simulink model "LM_TOS_0115"  (R2018b)
settings: Solver=FixedStepDiscrete  StartTime=0.0  StopTime=inf  FixedStep=0.005  RelTol=1e-3
PostLoadFcn:
  | if any(exist('dsrtsu_mdlpostloadfcn', 'file') ~= 0), dsrtsu_mdlpostloadfcn('Execute', bdroot); end
(part 2 of 4)

== system LM_TOS_0115/adapter2/HWA_TAR_OBJ_ADP/Subsystem4 ==
  <target_object_adapter> : Inport
  Bus Creator1 : BusCreator  Inputs=9  OutDataTypeStr=Bus: TARGETOBJECT  NonVirtualBus=on
  Bus Selector4 : BusSelector  OutputSignals=dis2EgoLaneCenter,TTC_f,ID_un8,Index_un8,probWithinLane_arr_f_0,probWithinLane_arr_f_1,probWithinLane_arr_f_2,probWithinLane_arr_f_3,probWithinLane_arr_f_4,probCutIn_f,probCutOut_f,overlap_f,trackingTimeWithinLane_f
  Vector Concatenate : Concatenate  NumInputs=5
  TARGRTOBJECTS_ST : Outport  OutDataTypeStr=Bus: TARGETOBJECT
  wires:
  Bus Selector4/8 -> Vector Concatenate/4  "<probWithinLane_arr_f_3>"
  Bus Selector4/11 -> Bus Creator1/7  "<probCutOut_f>"
  Bus Selector4/10 -> Bus Creator1/6  "<probCutIn_f>"
  Bus Selector4/12 -> Bus Creator1/8  "<overlap_f>"
  Bus Selector4/9 -> Vector Concatenate/5  "<probWithinLane_arr_f_4>"
  Bus Selector4/2 -> Bus Creator1/2  "<TTC_f>"
  Bus Selector4/5 -> Vector Concatenate/1  "<probWithinLane_arr_f_0>"
  <target_object_adapter>/1 -> Bus Selector4/1
  Bus Selector4/6 -> Vector Concatenate/2  "<probWithinLane_arr_f_1>"
  Bus Selector4/13 -> Bus Creator1/9  "<trackingTimeWithinLane_f>"
  Bus Selector4/1 -> Bus Creator1/1  "<dis2EgoLaneCenter>"
  Bus Selector4/7 -> Vector Concatenate/3  "<probWithinLane_arr_f_2>"
  Vector Concatenate/1 -> Bus Creator1/5
  Bus Selector4/3 -> Bus Creator1/3  "<ID_un8>"
  Bus Creator1/1 -> TARGRTOBJECTS_ST/1
  Bus Selector4/4 -> Bus Creator1/4  "<Index_un8>"

== system LM_TOS_0115/adapter2/HWA_TAR_OBJ_ADP/Subsystem5 ==
  <target_object_adapter> : Inport
  Bus Creator1 : BusCreator  Inputs=9  OutDataTypeStr=Bus: TARGETOBJECT  NonVirtualBus=on
  Bus Selector4 : BusSelector  OutputSignals=dis2EgoLaneCenter,TTC_f,ID_un8,Index_un8,probWithinLane_arr_f_0,probWithinLane_arr_f_1,probWithinLane_arr_f_2,probWithinLane_arr_f_3,probWithinLane_arr_f_4,probCutIn_f,probCutOut_f,overlap_f,trackingTimeWithinLane_f
  Vector Concatenate : Concatenate  NumInputs=5
  TARGRTOBJECTS_ST : Outport  OutDataTypeStr=Bus: TARGETOBJECT
  wires:
  Bus Selector4/4 -> Bus Creator1/4  "<Index_un8>"
  Bus Creator1/1 -> TARGRTOBJECTS_ST/1
  Bus Selector4/3 -> Bus Creator1/3  "<ID_un8>"
  Vector Concatenate/1 -> Bus Creator1/5
  Bus Selector4/7 -> Vector Concatenate/3  "<probWithinLane_arr_f_2>"
  Bus Selector4/1 -> Bus Creator1/1  "<dis2EgoLaneCenter>"
  Bus Selector4/13 -> Bus Creator1/9  "<trackingTimeWithinLane_f>"
  Bus Selector4/6 -> Vector Concatenate/2  "<probWithinLane_arr_f_1>"
  <target_object_adapter>/1 -> Bus Selector4/1
  Bus Selector4/5 -> Vector Concatenate/1  "<probWithinLane_arr_f_0>"
  Bus Selector4/2 -> Bus Creator1/2  "<TTC_f>"
  Bus Selector4/9 -> Vector Concatenate/5  "<probWithinLane_arr_f_4>"
  Bus Selector4/12 -> Bus Creator1/8  "<overlap_f>"
  Bus Selector4/10 -> Bus Creator1/6  "<probCutIn_f>"
  Bus Selector4/11 -> Bus Creator1/7  "<probCutOut_f>"
  Bus Selector4/8 -> Vector Concatenate/4  "<probWithinLane_arr_f_3>"

== system LM_TOS_0115/adapter2/HWA_TAR_OBJ_ADP/Subsystem6 ==
  <target_object_adapter> : Inport
  Bus Creator1 : BusCreator  Inputs=9  OutDataTypeStr=Bus: TARGETOBJECT  NonVirtualBus=on
  Bus Selector4 : BusSelector  OutputSignals=dis2EgoLaneCenter,TTC_f,ID_un8,Index_un8,probWithinLane_arr_f_0,probWithinLane_arr_f_1,probWithinLane_arr_f_2,probWithinLane_arr_f_3,probWithinLane_arr_f_4,probCutIn_f,probCutOut_f,overlap_f,trackingTimeWithinLane_f
  Vector Concatenate : Concatenate  NumInputs=5
  TARGRTOBJECTS_ST : Outport  OutDataTypeStr=Bus: TARGETOBJECT
  wires:
  Bus Selector4/8 -> Vector Concatenate/4  "<probWithinLane_arr_f_3>"
  Bus Selector4/11 -> Bus Creator1/7  "<probCutOut_f>"
  Bus Selector4/10 -> Bus Creator1/6  "<probCutIn_f>"
  Bus Selector4/12 -> Bus Creator1/8  "<overlap_f>"
  Bus Selector4/9 -> Vector Concatenate/5  "<probWithinLane_arr_f_4>"
  Bus Selector4/2 -> Bus Creator1/2  "<TTC_f>"
  Bus Selector4/5 -> Vector Concatenate/1  "<probWithinLane_arr_f_0>"
  <target_object_adapter>/1 -> Bus Selector4/1
  Bus Selector4/6 -> Vector Concatenate/2  "<probWithinLane_arr_f_1>"
  Bus Selector4/13 -> Bus Creator1/9  "<trackingTimeWithinLane_f>"
  Bus Selector4/1 -> Bus Creator1/1  "<dis2EgoLaneCenter>"
  Bus Selector4/7 -> Vector Concatenate/3  "<probWithinLane_arr_f_2>"
  Vector Concatenate/1 -> Bus Creator1/5
  Bus Selector4/3 -> Bus Creator1/3  "<ID_un8>"
  Bus Creator1/1 -> TARGRTOBJECTS_ST/1
  Bus Selector4/4 -> Bus Creator1/4  "<Index_un8>"

== system LM_TOS_0115/adapter2/HWA_TAR_OBJ_ADP/Subsystem7 ==
  <target_object_adapter> : Inport
  Bus Creator1 : BusCreator  Inputs=9  OutDataTypeStr=Bus: TARGETOBJECT  NonVirtualBus=on
  Bus Selector4 : BusSelector  OutputSignals=dis2EgoLaneCenter,TTC_f,ID_un8,Index_un8,probWithinLane_arr_f_0,probWithinLane_arr_f_1,probWithinLane_arr_f_2,probWithinLane_arr_f_3,probWithinLane_arr_f_4,probCutIn_f,probCutOut_f,overlap_f,trackingTimeWithinLane_f
  Vector Concatenate : Concatenate  NumInputs=5
  TARGRTOBJECTS_ST : Outport  OutDataTypeStr=Bus: TARGETOBJECT
  wires:
  Bus Selector4/4 -> Bus Creator1/4  "<Index_un8>"
  Bus Creator1/1 -> TARGRTOBJECTS_ST/1
  Bus Selector4/3 -> Bus Creator1/3  "<ID_un8>"
  Vector Concatenate/1 -> Bus Creator1/5
  Bus Selector4/7 -> Vector Concatenate/3  "<probWithinLane_arr_f_2>"
  Bus Selector4/1 -> Bus Creator1/1  "<dis2EgoLaneCenter>"
  Bus Selector4/13 -> Bus Creator1/9  "<trackingTimeWithinLane_f>"
  Bus Selector4/6 -> Vector Concatenate/2  "<probWithinLane_arr_f_1>"
  <target_object_adapter>/1 -> Bus Selector4/1
  Bus Selector4/5 -> Vector Concatenate/1  "<probWithinLane_arr_f_0>"
  Bus Selector4/2 -> Bus Creator1/2  "<TTC_f>"
  Bus Selector4/9 -> Vector Concatenate/5  "<probWithinLane_arr_f_4>"
  Bus Selector4/12 -> Bus Creator1/8  "<overlap_f>"
  Bus Selector4/10 -> Bus Creator1/6  "<probCutIn_f>"
  Bus Selector4/11 -> Bus Creator1/7  "<probCutOut_f>"
  Bus Selector4/8 -> Vector Concatenate/4  "<probWithinLane_arr_f_3>"

== system LM_TOS_0115/adapter2/HWA_TAR_OBJ_ADP/Subsystem8 ==
  <target_object_adapter> : Inport
  Bus Creator1 : BusCreator  Inputs=9  OutDataTypeStr=Bus: TARGETOBJECT  NonVirtualBus=on
  Bus Selector4 : BusSelector  OutputSignals=dis2EgoLaneCenter,TTC_f,ID_un8,Index_un8,probWithinLane_arr_f_0,probWithinLane_arr_f_1,probWithinLane_arr_f_2,probWithinLane_arr_f_3,probWithinLane_arr_f_4,probCutIn_f,probCutOut_f,overlap_f,trackingTimeWithinLane_f
  Vector Concatenate : Concatenate  NumInputs=5
  TARGRTOBJECTS_ST : Outport  OutDataTypeStr=Bus: TARGETOBJECT
  wires:
  Bus Selector4/8 -> Vector Concatenate/4  "<probWithinLane_arr_f_3>"
  Bus Selector4/11 -> Bus Creator1/7  "<probCutOut_f>"
  Bus Selector4/10 -> Bus Creator1/6  "<probCutIn_f>"
  Bus Selector4/12 -> Bus Creator1/8  "<overlap_f>"
  Bus Selector4/9 -> Vector Concatenate/5  "<probWithinLane_arr_f_4>"
  Bus Selector4/2 -> Bus Creator1/2  "<TTC_f>"
  Bus Selector4/5 -> Vector Concatenate/1  "<probWithinLane_arr_f_0>"
  <target_object_adapter>/1 -> Bus Selector4/1
  Bus Selector4/6 -> Vector Concatenate/2  "<probWithinLane_arr_f_1>"
  Bus Selector4/13 -> Bus Creator1/9  "<trackingTimeWithinLane_f>"
  Bus Selector4/1 -> Bus Creator1/1  "<dis2EgoLaneCenter>"
  Bus Selector4/7 -> Vector Concatenate/3  "<probWithinLane_arr_f_2>"
  Vector Concatenate/1 -> Bus Creator1/5
  Bus Selector4/3 -> Bus Creator1/3  "<ID_un8>"
  Bus Creator1/1 -> TARGRTOBJECTS_ST/1
  Bus Selector4/4 -> Bus Creator1/4  "<Index_un8>"

== system LM_TOS_0115/adapter2/HWA_TAR_OBJ_ADP/Subsystem9 ==
  <target_object_adapter> : Inport
  Bus Creator1 : BusCreator  Inputs=9  OutDataTypeStr=Bus: TARGETOBJECT  NonVirtualBus=on
  Bus Selector4 : BusSelector  OutputSignals=dis2EgoLaneCenter,TTC_f,ID_un8,Index_un8,probWithinLane_arr_f_0,probWithinLane_arr_f_1,probWithinLane_arr_f_2,probWithinLane_arr_f_3,probWithinLane_arr_f_4,probCutIn_f,probCutOut_f,overlap_f,trackingTimeWithinLane_f
  Vector Concatenate : Concatenate  NumInputs=5
  TARGRTOBJECTS_ST : Outport  OutDataTypeStr=Bus: TARGETOBJECT
  wires:
  Bus Selector4/4 -> Bus Creator1/4  "<Index_un8>"
  Bus Creator1/1 -> TARGRTOBJECTS_ST/1
  Bus Selector4/3 -> Bus Creator1/3  "<ID_un8>"
  Vector Concatenate/1 -> Bus Creator1/5
  Bus Selector4/7 -> Vector Concatenate/3  "<probWithinLane_arr_f_2>"
  Bus Selector4/1 -> Bus Creator1/1  "<dis2EgoLaneCenter>"
  Bus Selector4/13 -> Bus Creator1/9  "<trackingTimeWithinLane_f>"
  Bus Selector4/6 -> Vector Concatenate/2  "<probWithinLane_arr_f_1>"
  <target_object_adapter>/1 -> Bus Selector4/1
  Bus Selector4/5 -> Vector Concatenate/1  "<probWithinLane_arr_f_0>"
  Bus Selector4/2 -> Bus Creator1/2  "<TTC_f>"
  Bus Selector4/9 -> Vector Concatenate/5  "<probWithinLane_arr_f_4>"
  Bus Selector4/12 -> Bus Creator1/8  "<overlap_f>"
  Bus Selector4/10 -> Bus Creator1/6  "<probCutIn_f>"
  Bus Selector4/11 -> Bus Creator1/7  "<probCutOut_f>"
  Bus Selector4/8 -> Vector Concatenate/4  "<probWithinLane_arr_f_3>"

== system LM_TOS_0115/adapter2/Lane_0/Subsystem ==
  <LANE_0_TARGETOBJECT_0_ST> : Inport
  Bus Creator1 : BusCreator  Inputs=9  OutDataTypeStr=Bus: TARGETOBJECT  NonVirtualBus=on
  Bus Selector4 : BusSelector  OutputSignals=dis2EgoLaneCenter,TTC_f,ID_un8,Index_un8,probWithinLane_arr_f_0,probWithinLane_arr_f_1,probWithinLane_arr_f_2,probWithinLane_arr_f_3,probWithinLane_arr_f_4,probCutIn_f,probCutOut_f,overlap_f,trackingTimeWithinLane_f
  Vector Concatenate : Concatenate  NumInputs=5
  TARGRTOBJECTS_ST : Outport  OutDataTypeStr=Bus: TARGETOBJECT
  wires:
  Bus Selector4/4 -> Bus Creator1/4  "<Index_un8>"
  Bus Creator1/1 -> TARGRTOBJECTS_ST/1
  Bus Selector4/3 -> Bus Creator1/3  "<ID_un8>"
  Vector Concatenate/1 -> Bus Creator1/5
  Bus Selector4/7 -> Vector Concatenate/3  "<probWithinLane_arr_f_2>"
  Bus Selector4/1 -> Bus Creator1/1  "<dis2EgoLaneCenter>"
  Bus Selector4/13 -> Bus Creator1/9  "<trackingTimeWithinLane_f>"
  Bus Selector4/6 -> Vector Concatenate/2  "<probWithinLane_arr_f_1>"
  <LANE_0_TARGETOBJECT_0_ST>/1 -> Bus Selector4/1
  Bus Selector4/5 -> Vector Concatenate/1  "<probWithinLane_arr_f_0>"
  Bus Selector4/2 -> Bus Creator1/2  "<TTC_f>"
  Bus Selector4/9 -> Vector Concatenate/5  "<probWithinLane_arr_f_4>"
  Bus Selector4/12 -> Bus Creator1/8  "<overlap_f>"
  Bus Selector4/10 -> Bus Creator1/6  "<probCutIn_f>"
  Bus Selector4/11 -> Bus Creator1/7  "<probCutOut_f>"
  Bus Selector4/8 -> Vector Concatenate/4  "<probWithinLane_arr_f_3>"

== system LM_TOS_0115/adapter2/Lane_0/Subsystem1 ==
  <LANE_0_TARGETOBJECT_0_ST> : Inport
  Bus Creator1 : BusCreator  Inputs=9  OutDataTypeStr=Bus: TARGETOBJECT  NonVirtualBus=on
  Bus Selector4 : BusSelector  OutputSignals=dis2EgoLaneCenter,TTC_f,ID_un8,Index_un8,probWithinLane_arr_f_0,probWithinLane_arr_f_1,probWithinLane_arr_f_2,probWithinLane_arr_f_3,probWithinLane_arr_f_4,probCutIn_f,probCutOut_f,overlap_f,trackingTimeWithinLane_f
  Vector Concatenate : Concatenate  NumInputs=5
  TARGRTOBJECTS_ST : Outport  OutDataTypeStr=Bus: TARGETOBJECT
  wires:
  Bus Selector4/8 -> Vector Concatenate/4  "<probWithinLane_arr_f_3>"
  Bus Selector4/11 -> Bus Creator1/7  "<probCutOut_f>"
  Bus Selector4/10 -> Bus Creator1/6  "<probCutIn_f>"
  Bus Selector4/12 -> Bus Creator1/8  "<overlap_f>"
  Bus Selector4/9 -> Vector Concatenate/5  "<probWithinLane_arr_f_4>"
  Bus Selector4/2 -> Bus Creator1/2  "<TTC_f>"
  Bus Selector4/5 -> Vector Concatenate/1  "<probWithinLane_arr_f_0>"
  <LANE_0_TARGETOBJECT_0_ST>/1 -> Bus Selector4/1
  Bus Selector4/6 -> Vector Concatenate/2  "<probWithinLane_arr_f_1>"
  Bus Selector4/13 -> Bus Creator1/9  "<trackingTimeWithinLane_f>"
  Bus Selector4/1 -> Bus Creator1/1  "<dis2EgoLaneCenter>"
  Bus Selector4/7 -> Vector Concatenate/3  "<probWithinLane_arr_f_2>"
  Vector Concatenate/1 -> Bus Creator1/5
  Bus Selector4/3 -> Bus Creator1/3  "<ID_un8>"
  Bus Creator1/1 -> TARGRTOBJECTS_ST/1
  Bus Selector4/4 -> Bus Creator1/4  "<Index_un8>"

== system LM_TOS_0115/adapter2/Lane_0/Subsystem10 ==
  <LANE_0_TARGETOBJECT_0_ST> : Inport
  Bus Creator1 : BusCreator  Inputs=7  OutDataTypeStr=Bus: SEGMENT  NonVirtualBus=on
  Bus Selector4 : BusSelector  OutputSignals=coef_arr_f_0,coef_arr_f_1,coef_arr_f_2,coef_arr_f_3,dlowerLimit_f,dupperLimit_f,numOfSegment_un8,available_b,detectedByVideo_b,quality_f
  Vector Concatenate : Concatenate  NumInputs=4
  SEGMENT_ST : Outport  OutDataTypeStr=Bus: SEGMENT
  wires:
  Bus Creator1/1 -> SEGMENT_ST/1
  <LANE_0_TARGETOBJECT_0_ST>/1 -> Bus Selector4/1
  Bus Selector4/2 -> Vector Concatenate/2  "<coef_arr_f_1>"
  Bus Selector4/1 -> Vector Concatenate/1  "<coef_arr_f_0>"
  Bus Selector4/3 -> Vector Concatenate/3  "<coef_arr_f_2>"
  Bus Selector4/4 -> Vector Concatenate/4  "<coef_arr_f_3>"
  Vector Concatenate/1 -> Bus Creator1/1
  Bus Selector4/5 -> Bus Creator1/2  "<dlowerLimit_f>"
  Bus Selector4/10 -> Bus Creator1/7  "<quality_f>"
  Bus Selector4/9 -> Bus Creator1/6  "<detectedByVideo_b>"
  Bus Selector4/8 -> Bus Creator1/5  "<available_b>"
  Bus Selector4/7 -> Bus Creator1/4  "<numOfSegment_un8>"
  Bus Selector4/6 -> Bus Creator1/3  "<dupperLimit_f>"

== system LM_TOS_0115/adapter2/Lane_0/Subsystem11 ==
  <LANE_0_TARGETOBJECT_0_ST> : Inport
  Bus Creator1 : BusCreator  Inputs=7  OutDataTypeStr=Bus: SEGMENT  NonVirtualBus=on
  Bus Selector4 : BusSelector  OutputSignals=coef_arr_f_0,coef_arr_f_1,coef_arr_f_2,coef_arr_f_3,dlowerLimit_f,dupperLimit_f,numOfSegment_un8,available_b,detectedByVideo_b,quality_f
  Vector Concatenate : Concatenate  NumInputs=4
  SEGMENT_ST : Outport  OutDataTypeStr=Bus: SEGMENT
  wires:
  Bus Selector4/6 -> Bus Creator1/3  "<dupperLimit_f>"
  Bus Selector4/7 -> Bus Creator1/4  "<numOfSegment_un8>"
  Bus Selector4/8 -> Bus Creator1/5  "<available_b>"
  Bus Selector4/9 -> Bus Creator1/6  "<detectedByVideo_b>"
  Bus Selector4/10 -> Bus Creator1/7  "<quality_f>"
  Bus Selector4/5 -> Bus Creator1/2  "<dlowerLimit_f>"
  Vector Concatenate/1 -> Bus Creator1/1
  Bus Selector4/4 -> Vector Concatenate/4  "<coef_arr_f_3>"
  Bus Selector4/3 -> Vector Concatenate/3  "<coef_arr_f_2>"
  Bus Selector4/1 -> Vector Concatenate/1  "<coef_arr_f_0>"
  Bus Selector4/2 -> Vector Concatenate/2  "<coef_arr_f_1>"
  <LANE_0_TARGETOBJECT_0_ST>/1 -> Bus Selector4/1
  Bus Creator1/1 -> SEGMENT_ST/1

== system LM_TOS_0115/adapter2/Lane_0/Subsystem12 ==
  <LANE_0_TARGETOBJECT_0_ST> : Inport
  Bus Creator1 : BusCreator  Inputs=7  OutDataTypeStr=Bus: SEGMENT  NonVirtualBus=on
  Bus Selector4 : BusSelector  OutputSignals=coef_arr_f_0,coef_arr_f_1,coef_arr_f_2,coef_arr_f_3,dlowerLimit_f,dupperLimit_f,numOfSegment_un8,available_b,detectedByVideo_b,quality_f
  Vector Concatenate : Concatenate  NumInputs=4
  SEGMENT_ST : Outport  OutDataTypeStr=Bus: SEGMENT
  wires:
  Bus Creator1/1 -> SEGMENT_ST/1
  <LANE_0_TARGETOBJECT_0_ST>/1 -> Bus Selector4/1
  Bus Selector4/2 -> Vector Concatenate/2  "<coef_arr_f_1>"
  Bus Selector4/1 -> Vector Concatenate/1  "<coef_arr_f_0>"
  Bus Selector4/3 -> Vector Concatenate/3  "<coef_arr_f_2>"
  Bus Selector4/4 -> Vector Concatenate/4  "<coef_arr_f_3>"
  Vector Concatenate/1 -> Bus Creator1/1
  Bus Selector4/5 -> Bus Creator1/2  "<dlowerLimit_f>"
  Bus Selector4/10 -> Bus Creator1/7  "<quality_f>"
  Bus Selector4/9 -> Bus Creator1/6  "<detectedByVideo_b>"
  Bus Selector4/8 -> Bus Creator1/5  "<available_b>"
  Bus Selector4/7 -> Bus Creator1/4  "<numOfSegment_un8>"
  Bus Selector4/6 -> Bus Creator1/3  "<dupperLimit_f>"

== system LM_TOS_0115/adapter2/Lane_0/Subsystem13 ==
  <LANE_0_TARGETOBJECT_0_ST> : Inport
  Bus Creator1 : BusCreator  Inputs=7  OutDataTypeStr=Bus: SEGMENT  NonVirtualBus=on
  Bus Selector4 : BusSelector  OutputSignals=coef_arr_f_0,coef_arr_f_1,coef_arr_f_2,coef_arr_f_3,dlowerLimit_f,dupperLimit_f,numOfSegment_un8,available_b,detectedByVideo_b,quality_f
  Vector Concatenate : Concatenate  NumInputs=4
  SEGMENT_ST : Outport  OutDataTypeStr=Bus: SEGMENT
  wires:
  Bus Selector4/6 -> Bus Creator1/3  "<dupperLimit_f>"
  Bus Selector4/7 -> Bus Creator1/4  "<numOfSegment_un8>"
  Bus Selector4/8 -> Bus Creator1/5  "<available_b>"
  Bus Selector4/9 -> Bus Creator1/6  "<detectedByVideo_b>"
  Bus Selector4/10 -> Bus Creator1/7  "<quality_f>"
  Bus Selector4/5 -> Bus Creator1/2  "<dlowerLimit_f>"
  Vector Concatenate/1 -> Bus Creator1/1
  Bus Selector4/4 -> Vector Concatenate/4  "<coef_arr_f_3>"
  Bus Selector4/3 -> Vector Concatenate/3  "<coef_arr_f_2>"
  Bus Selector4/1 -> Vector Concatenate/1  "<coef_arr_f_0>"
  Bus Selector4/2 -> Vector Concatenate/2  "<coef_arr_f_1>"
  <LANE_0_TARGETOBJECT_0_ST>/1 -> Bus Selector4/1
  Bus Creator1/1 -> SEGMENT_ST/1

== system LM_TOS_0115/adapter2/Lane_0/Subsystem14 ==
  <LANE_0_TARGETOBJECT_0_ST> : Inport
  Bus Creator1 : BusCreator  Inputs=7  OutDataTypeStr=Bus: SEGMENT  NonVirtualBus=on
  Bus Selector4 : BusSelector  OutputSignals=coef_arr_f_0,coef_arr_f_1,coef_arr_f_2,coef_arr_f_3,dlowerLimit_f,dupperLimit_f,numOfSegment_un8,available_b,detectedByVideo_b,quality_f
  Vector Concatenate : Concatenate  NumInputs=4
  SEGMENT_ST : Outport  OutDataTypeStr=Bus: SEGMENT
  wires:
  Bus Creator1/1 -> SEGMENT_ST/1
  <LANE_0_TARGETOBJECT_0_ST>/1 -> Bus Selector4/1
  Bus Selector4/2 -> Vector Concatenate/2  "<coef_arr_f_1>"
  Bus Selector4/1 -> Vector Concatenate/1  "<coef_arr_f_0>"
  Bus Selector4/3 -> Vector Concatenate/3  "<coef_arr_f_2>"
  Bus Selector4/4 -> Vector Concatenate/4  "<coef_arr_f_3>"
  Vector Concatenate/1 -> Bus Creator1/1
  Bus Selector4/5 -> Bus Creator1/2  "<dlowerLimit_f>"
  Bus Selector4/10 -> Bus Creator1/7  "<quality_f>"
  Bus Selector4/9 -> Bus Creator1/6  "<detectedByVideo_b>"
  Bus Selector4/8 -> Bus Creator1/5  "<available_b>"
  Bus Selector4/7 -> Bus Creator1/4  "<numOfSegment_un8>"
  Bus Selector4/6 -> Bus Creator1/3  "<dupperLimit_f>"

== system LM_TOS_0115/adapter2/Lane_0/Subsystem15 ==
  <LANE_0_TARGETOBJECT_0_ST> : Inport
  Bus Creator1 : BusCreator  Inputs=7  OutDataTypeStr=Bus: SEGMENT  NonVirtualBus=on
  Bus Selector4 : BusSelector  OutputSignals=coef_arr_f_0,coef_arr_f_1,coef_arr_f_2,coef_arr_f_3,dlowerLimit_f,dupperLimit_f,numOfSegment_un8,available_b,detectedByVideo_b,quality_f
  Vector Concatenate : Concatenate  NumInputs=4
  SEGMENT_ST : Outport  OutDataTypeStr=Bus: SEGMENT
  wires:
  Bus Selector4/6 -> Bus Creator1/3  "<dupperLimit_f>"
  Bus Selector4/7 -> Bus Creator1/4  "<numOfSegment_un8>"
  Bus Selector4/8 -> Bus Creator1/5  "<available_b>"
  Bus Selector4/9 -> Bus Creator1/6  "<detectedByVideo_b>"
  Bus Selector4/10 -> Bus Creator1/7  "<quality_f>"
  Bus Selector4/5 -> Bus Creator1/2  "<dlowerLimit_f>"
  Vector Concatenate/1 -> Bus Creator1/1
  Bus Selector4/4 -> Vector Concatenate/4  "<coef_arr_f_3>"
  Bus Selector4/3 -> Vector Concatenate/3  "<coef_arr_f_2>"
  Bus Selector4/1 -> Vector Concatenate/1  "<coef_arr_f_0>"
  Bus Selector4/2 -> Vector Concatenate/2  "<coef_arr_f_1>"
  <LANE_0_TARGETOBJECT_0_ST>/1 -> Bus Selector4/1
  Bus Creator1/1 -> SEGMENT_ST/1

== system LM_TOS_0115/adapter2/Lane_0/Subsystem2 ==
  <LANE_0_TARGETOBJECT_0_ST> : Inport
  Bus Creator1 : BusCreator  Inputs=9  OutDataTypeStr=Bus: TARGETOBJECT  NonVirtualBus=on
  Bus Selector4 : BusSelector  OutputSignals=dis2EgoLaneCenter,TTC_f,ID_un8,Index_un8,probWithinLane_arr_f_0,probWithinLane_arr_f_1,probWithinLane_arr_f_2,probWithinLane_arr_f_3,probWithinLane_arr_f_4,probCutIn_f,probCutOut_f,overlap_f,trackingTimeWithinLane_f
  Vector Concatenate : Concatenate  NumInputs=5
  TARGRTOBJECTS_ST : Outport  OutDataTypeStr=Bus: TARGETOBJECT
  wires:
  Bus Selector4/4 -> Bus Creator1/4  "<Index_un8>"
  Bus Creator1/1 -> TARGRTOBJECTS_ST/1
  Bus Selector4/3 -> Bus Creator1/3  "<ID_un8>"
  Vector Concatenate/1 -> Bus Creator1/5
  Bus Selector4/7 -> Vector Concatenate/3  "<probWithinLane_arr_f_2>"
  Bus Selector4/1 -> Bus Creator1/1  "<dis2EgoLaneCenter>"
  Bus Selector4/13 -> Bus Creator1/9  "<trackingTimeWithinLane_f>"
  Bus Selector4/6 -> Vector Concatenate/2  "<probWithinLane_arr_f_1>"
  <LANE_0_TARGETOBJECT_0_ST>/1 -> Bus Selector4/1
  Bus Selector4/5 -> Vector Concatenate/1  "<probWithinLane_arr_f_0>"
  Bus Selector4/2 -> Bus Creator1/2  "<TTC_f>"
  Bus Selector4/9 -> Vector Concatenate/5  "<probWithinLane_arr_f_4>"
  Bus Selector4/12 -> Bus Creator1/8  "<overlap_f>"
  Bus Selector4/10 -> Bus Creator1/6  "<probCutIn_f>"
  Bus Selector4/11 -> Bus Creator1/7  "<probCutOut_f>"
  Bus Selector4/8 -> Vector Concatenate/4  "<probWithinLane_arr_f_3>"

== system LM_TOS_0115/adapter2/Lane_0/Subsystem3 ==
  <LANE_0_TARGETOBJECT_0_ST> : Inport
  Bus Creator1 : BusCreator  Inputs=9  OutDataTypeStr=Bus: TARGETOBJECT  NonVirtualBus=on
  Bus Selector4 : BusSelector  OutputSignals=dis2EgoLaneCenter,TTC_f,ID_un8,Index_un8,probWithinLane_arr_f_0,probWithinLane_arr_f_1,probWithinLane_arr_f_2,probWithinLane_arr_f_3,probWithinLane_arr_f_4,probCutIn_f,probCutOut_f,overlap_f,trackingTimeWithinLane_f
  Vector Concatenate : Concatenate  NumInputs=5
  TARGRTOBJECTS_ST : Outport  OutDataTypeStr=Bus: TARGETOBJECT
  wires:
  Bus Selector4/8 -> Vector Concatenate/4  "<probWithinLane_arr_f_3>"
  Bus Selector4/11 -> Bus Creator1/7  "<probCutOut_f>"
  Bus Selector4/10 -> Bus Creator1/6  "<probCutIn_f>"
  Bus Selector4/12 -> Bus Creator1/8  "<overlap_f>"
  Bus Selector4/9 -> Vector Concatenate/5  "<probWithinLane_arr_f_4>"
  Bus Selector4/2 -> Bus Creator1/2  "<TTC_f>"
  Bus Selector4/5 -> Vector Concatenate/1  "<probWithinLane_arr_f_0>"
  <LANE_0_TARGETOBJECT_0_ST>/1 -> Bus Selector4/1
  Bus Selector4/6 -> Vector Concatenate/2  "<probWithinLane_arr_f_1>"
  Bus Selector4/13 -> Bus Creator1/9  "<trackingTimeWithinLane_f>"
  Bus Selector4/1 -> Bus Creator1/1  "<dis2EgoLaneCenter>"
  Bus Selector4/7 -> Vector Concatenate/3  "<probWithinLane_arr_f_2>"
  Vector Concatenate/1 -> Bus Creator1/5
  Bus Selector4/3 -> Bus Creator1/3  "<ID_un8>"
  Bus Creator1/1 -> TARGRTOBJECTS_ST/1
  Bus Selector4/4 -> Bus Creator1/4  "<Index_un8>"

== system LM_TOS_0115/adapter2/Lane_0/Subsystem4 ==
  <LANE_0_TARGETOBJECT_0_ST> : Inport
  Bus Creator1 : BusCreator  Inputs=9  OutDataTypeStr=Bus: TARGETOBJECT  NonVirtualBus=on
  Bus Selector4 : BusSelector  OutputSignals=dis2EgoLaneCenter,TTC_f,ID_un8,Index_un8,probWithinLane_arr_f_0,probWithinLane_arr_f_1,probWithinLane_arr_f_2,probWithinLane_arr_f_3,probWithinLane_arr_f_4,probCutIn_f,probCutOut_f,overlap_f,trackingTimeWithinLane_f
  Vector Concatenate : Concatenate  NumInputs=5
  TARGRTOBJECTS_ST : Outport  OutDataTypeStr=Bus: TARGETOBJECT
  wires:
  Bus Selector4/4 -> Bus Creator1/4  "<Index_un8>"
  Bus Creator1/1 -> TARGRTOBJECTS_ST/1
  Bus Selector4/3 -> Bus Creator1/3  "<ID_un8>"
  Vector Concatenate/1 -> Bus Creator1/5
  Bus Selector4/7 -> Vector Concatenate/3  "<probWithinLane_arr_f_2>"
  Bus Selector4/1 -> Bus Creator1/1  "<dis2EgoLaneCenter>"
  Bus Selector4/13 -> Bus Creator1/9  "<trackingTimeWithinLane_f>"
  Bus Selector4/6 -> Vector Concatenate/2  "<probWithinLane_arr_f_1>"
  <LANE_0_TARGETOBJECT_0_ST>/1 -> Bus Selector4/1
  Bus Selector4/5 -> Vector Concatenate/1  "<probWithinLane_arr_f_0>"
  Bus Selector4/2 -> Bus Creator1/2  "<TTC_f>"
  Bus Selector4/9 -> Vector Concatenate/5  "<probWithinLane_arr_f_4>"
  Bus Selector4/12 -> Bus Creator1/8  "<overlap_f>"
  Bus Selector4/10 -> Bus Creator1/6  "<probCutIn_f>"
  Bus Selector4/11 -> Bus Creator1/7  "<probCutOut_f>"
  Bus Selector4/8 -> Vector Concatenate/4  "<probWithinLane_arr_f_3>"

== system LM_TOS_0115/adapter2/Lane_0/Subsystem5 ==
  <LANE_0_TARGETOBJECT_0_ST> : Inport
  Bus Creator1 : BusCreator  Inputs=9  OutDataTypeStr=Bus: TARGETOBJECT  NonVirtualBus=on
  Bus Selector4 : BusSelector  OutputSignals=dis2EgoLaneCenter,TTC_f,ID_un8,Index_un8,probWithinLane_arr_f_0,probWithinLane_arr_f_1,probWithinLane_arr_f_2,probWithinLane_arr_f_3,probWithinLane_arr_f_4,probCutIn_f,probCutOut_f,overlap_f,trackingTimeWithinLane_f
  Vector Concatenate : Concatenate  NumInputs=5
  TARGRTOBJECTS_ST : Outport  OutDataTypeStr=Bus: TARGETOBJECT
  wires:
  Bus Selector4/8 -> Vector Concatenate/4  "<probWithinLane_arr_f_3>"
  Bus Selector4/11 -> Bus Creator1/7  "<probCutOut_f>"
  Bus Selector4/10 -> Bus Creator1/6  "<probCutIn_f>"
  Bus Selector4/12 -> Bus Creator1/8  "<overlap_f>"
  Bus Selector4/9 -> Vector Concatenate/5  "<probWithinLane_arr_f_4>"
  Bus Selector4/2 -> Bus Creator1/2  "<TTC_f>"
  Bus Selector4/5 -> Vector Concatenate/1  "<probWithinLane_arr_f_0>"
  <LANE_0_TARGETOBJECT_0_ST>/1 -> Bus Selector4/1
  Bus Selector4/6 -> Vector Concatenate/2  "<probWithinLane_arr_f_1>"
  Bus Selector4/13 -> Bus Creator1/9  "<trackingTimeWithinLane_f>"
  Bus Selector4/1 -> Bus Creator1/1  "<dis2EgoLaneCenter>"
  Bus Selector4/7 -> Vector Concatenate/3  "<probWithinLane_arr_f_2>"
  Vector Concatenate/1 -> Bus Creator1/5
  Bus Selector4/3 -> Bus Creator1/3  "<ID_un8>"
  Bus Creator1/1 -> TARGRTOBJECTS_ST/1
  Bus Selector4/4 -> Bus Creator1/4  "<Index_un8>"

== system LM_TOS_0115/adapter2/Lane_0/Subsystem6 ==
  <LANE_0_TARGETOBJECT_0_ST> : Inport
  Bus Creator1 : BusCreator  Inputs=9  OutDataTypeStr=Bus: TARGETOBJECT  NonVirtualBus=on
  Bus Selector4 : BusSelector  OutputSignals=dis2EgoLaneCenter,TTC_f,ID_un8,Index_un8,probWithinLane_arr_f_0,probWithinLane_arr_f_1,probWithinLane_arr_f_2,probWithinLane_arr_f_3,probWithinLane_arr_f_4,probCutIn_f,probCutOut_f,overlap_f,trackingTimeWithinLane_f
  Vector Concatenate : Concatenate  NumInputs=5
  TARGRTOBJECTS_ST : Outport  OutDataTypeStr=Bus: TARGETOBJECT
  wires:
  Bus Selector4/4 -> Bus Creator1/4  "<Index_un8>"
  Bus Creator1/1 -> TARGRTOBJECTS_ST/1
  Bus Selector4/3 -> Bus Creator1/3  "<ID_un8>"
  Vector Concatenate/1 -> Bus Creator1/5
  Bus Selector4/7 -> Vector Concatenate/3  "<probWithinLane_arr_f_2>"
  Bus Selector4/1 -> Bus Creator1/1  "<dis2EgoLaneCenter>"
  Bus Selector4/13 -> Bus Creator1/9  "<trackingTimeWithinLane_f>"
  Bus Selector4/6 -> Vector Concatenate/2  "<probWithinLane_arr_f_1>"
  <LANE_0_TARGETOBJECT_0_ST>/1 -> Bus Selector4/1
  Bus Selector4/5 -> Vector Concatenate/1  "<probWithinLane_arr_f_0>"
  Bus Selector4/2 -> Bus Creator1/2  "<TTC_f>"
  Bus Selector4/9 -> Vector Concatenate/5  "<probWithinLane_arr_f_4>"
  Bus Selector4/12 -> Bus Creator1/8  "<overlap_f>"
  Bus Selector4/10 -> Bus Creator1/6  "<probCutIn_f>"
  Bus Selector4/11 -> Bus Creator1/7  "<probCutOut_f>"
  Bus Selector4/8 -> Vector Concatenate/4  "<probWithinLane_arr_f_3>"

== system LM_TOS_0115/adapter2/Lane_0/Subsystem7 ==
  <LANE_0_TARGETOBJECT_0_ST> : Inport
  Bus Creator1 : BusCreator  Inputs=9  OutDataTypeStr=Bus: TARGETOBJECT  NonVirtualBus=on
  Bus Selector4 : BusSelector  OutputSignals=dis2EgoLaneCenter,TTC_f,ID_un8,Index_un8,probWithinLane_arr_f_0,probWithinLane_arr_f_1,probWithinLane_arr_f_2,probWithinLane_arr_f_3,probWithinLane_arr_f_4,probCutIn_f,probCutOut_f,overlap_f,trackingTimeWithinLane_f
  Vector Concatenate : Concatenate  NumInputs=5
  TARGRTOBJECTS_ST : Outport  OutDataTypeStr=Bus: TARGETOBJECT
  wires:
  Bus Selector4/8 -> Vector Concatenate/4  "<probWithinLane_arr_f_3>"
  Bus Selector4/11 -> Bus Creator1/7  "<probCutOut_f>"
  Bus Selector4/10 -> Bus Creator1/6  "<probCutIn_f>"
  Bus Selector4/12 -> Bus Creator1/8  "<overlap_f>"
  Bus Selector4/9 -> Vector Concatenate/5  "<probWithinLane_arr_f_4>"
  Bus Selector4/2 -> Bus Creator1/2  "<TTC_f>"
  Bus Selector4/5 -> Vector Concatenate/1  "<probWithinLane_arr_f_0>"
  <LANE_0_TARGETOBJECT_0_ST>/1 -> Bus Selector4/1
  Bus Selector4/6 -> Vector Concatenate/2  "<probWithinLane_arr_f_1>"
  Bus Selector4/13 -> Bus Creator1/9  "<trackingTimeWithinLane_f>"
  Bus Selector4/1 -> Bus Creator1/1  "<dis2EgoLaneCenter>"
  Bus Selector4/7 -> Vector Concatenate/3  "<probWithinLane_arr_f_2>"
  Vector Concatenate/1 -> Bus Creator1/5
  Bus Selector4/3 -> Bus Creator1/3  "<ID_un8>"
  Bus Creator1/1 -> TARGRTOBJECTS_ST/1
  Bus Selector4/4 -> Bus Creator1/4  "<Index_un8>"

== system LM_TOS_0115/adapter2/Lane_0/Subsystem8 ==
  <LANE_0_TARGETOBJECT_0_ST> : Inport
  Bus Creator1 : BusCreator  Inputs=9  OutDataTypeStr=Bus: TARGETOBJECT  NonVirtualBus=on
  Bus Selector4 : BusSelector  OutputSignals=dis2EgoLaneCenter,TTC_f,ID_un8,Index_un8,probWithinLane_arr_f_0,probWithinLane_arr_f_1,probWithinLane_arr_f_2,probWithinLane_arr_f_3,probWithinLane_arr_f_4,probCutIn_f,probCutOut_f,overlap_f,trackingTimeWithinLane_f
  Vector Concatenate : Concatenate  NumInputs=5
  TARGRTOBJECTS_ST : Outport  OutDataTypeStr=Bus: TARGETOBJECT
  wires:
  Bus Selector4/4 -> Bus Creator1/4  "<Index_un8>"
  Bus Creator1/1 -> TARGRTOBJECTS_ST/1
  Bus Selector4/3 -> Bus Creator1/3  "<ID_un8>"
  Vector Concatenate/1 -> Bus Creator1/5
  Bus Selector4/7 -> Vector Concatenate/3  "<probWithinLane_arr_f_2>"
  Bus Selector4/1 -> Bus Creator1/1  "<dis2EgoLaneCenter>"
  Bus Selector4/13 -> Bus Creator1/9  "<trackingTimeWithinLane_f>"
  Bus Selector4/6 -> Vector Concatenate/2  "<probWithinLane_arr_f_1>"
  <LANE_0_TARGETOBJECT_0_ST>/1 -> Bus Selector4/1
  Bus Selector4/5 -> Vector Concatenate/1  "<probWithinLane_arr_f_0>"
  Bus Selector4/2 -> Bus Creator1/2  "<TTC_f>"
  Bus Selector4/9 -> Vector Concatenate/5  "<probWithinLane_arr_f_4>"
  Bus Selector4/12 -> Bus Creator1/8  "<overlap_f>"
  Bus Selector4/10 -> Bus Creator1/6  "<probCutIn_f>"
  Bus Selector4/11 -> Bus Creator1/7  "<probCutOut_f>"
  Bus Selector4/8 -> Vector Concatenate/4  "<probWithinLane_arr_f_3>"

== system LM_TOS_0115/adapter2/Lane_0/Subsystem9 ==
  <LANE_0_TARGETOBJECT_0_ST> : Inport
  Bus Creator1 : BusCreator  Inputs=9  OutDataTypeStr=Bus: TARGETOBJECT  NonVirtualBus=on
  Bus Selector4 : BusSelector  OutputSignals=dis2EgoLaneCenter,TTC_f,ID_un8,Index_un8,probWithinLane_arr_f_0,probWithinLane_arr_f_1,probWithinLane_arr_f_2,probWithinLane_arr_f_3,probWithinLane_arr_f_4,probCutIn_f,probCutOut_f,overlap_f,trackingTimeWithinLane_f
  Vector Concatenate : Concatenate  NumInputs=5
  TARGRTOBJECTS_ST : Outport  OutDataTypeStr=Bus: TARGETOBJECT
  wires:
  Bus Selector4/8 -> Vector Concatenate/4  "<probWithinLane_arr_f_3>"
  Bus Selector4/11 -> Bus Creator1/7  "<probCutOut_f>"
  Bus Selector4/10 -> Bus Creator1/6  "<probCutIn_f>"
  Bus Selector4/12 -> Bus Creator1/8  "<overlap_f>"
  Bus Selector4/9 -> Vector Concatenate/5  "<probWithinLane_arr_f_4>"
  Bus Selector4/2 -> Bus Creator1/2  "<TTC_f>"
  Bus Selector4/5 -> Vector Concatenate/1  "<probWithinLane_arr_f_0>"
  <LANE_0_TARGETOBJECT_0_ST>/1 -> Bus Selector4/1
  Bus Selector4/6 -> Vector Concatenate/2  "<probWithinLane_arr_f_1>"
  Bus Selector4/13 -> Bus Creator1/9  "<trackingTimeWithinLane_f>"
  Bus Selector4/1 -> Bus Creator1/1  "<dis2EgoLaneCenter>"
  Bus Selector4/7 -> Vector Concatenate/3  "<probWithinLane_arr_f_2>"
  Vector Concatenate/1 -> Bus Creator1/5
  Bus Selector4/3 -> Bus Creator1/3  "<ID_un8>"
  Bus Creator1/1 -> TARGRTOBJECTS_ST/1
  Bus Selector4/4 -> Bus Creator1/4  "<Index_un8>"

== system LM_TOS_0115/adapter2/Lane_1/Subsystem ==
  <LANE_1_TARGETOBJECT_0_ST> : Inport
  Bus Creator1 : BusCreator  Inputs=9  OutDataTypeStr=Bus: TARGETOBJECT  NonVirtualBus=on
  Bus Selector4 : BusSelector  OutputSignals=dis2EgoLaneCenter,TTC_f,ID_un8,Index_un8,probWithinLane_arr_f_0,probWithinLane_arr_f_1,probWithinLane_arr_f_2,probWithinLane_arr_f_3,probWithinLane_arr_f_4,probCutIn_f,probCutOut_f,overlap_f,trackingTimeWithinLane_f
  Vector Concatenate : Concatenate  NumInputs=5
  TARGRTOBJECTS_ST : Outport  OutDataTypeStr=Bus: TARGETOBJECT
  wires:
  Bus Selector4/8 -> Vector Concatenate/4  "<probWithinLane_arr_f_3>"
  Bus Selector4/11 -> Bus Creator1/7  "<probCutOut_f>"
  Bus Selector4/10 -> Bus Creator1/6  "<probCutIn_f>"
  Bus Selector4/12 -> Bus Creator1/8  "<overlap_f>"
  Bus Selector4/9 -> Vector Concatenate/5  "<probWithinLane_arr_f_4>"
  Bus Selector4/2 -> Bus Creator1/2  "<TTC_f>"
  Bus Selector4/5 -> Vector Concatenate/1  "<probWithinLane_arr_f_0>"
  <LANE_1_TARGETOBJECT_0_ST>/1 -> Bus Selector4/1
  Bus Selector4/6 -> Vector Concatenate/2  "<probWithinLane_arr_f_1>"
  Bus Selector4/13 -> Bus Creator1/9  "<trackingTimeWithinLane_f>"
  Bus Selector4/1 -> Bus Creator1/1  "<dis2EgoLaneCenter>"
  Bus Selector4/7 -> Vector Concatenate/3  "<probWithinLane_arr_f_2>"
  Vector Concatenate/1 -> Bus Creator1/5
  Bus Selector4/3 -> Bus Creator1/3  "<ID_un8>"
  Bus Creator1/1 -> TARGRTOBJECTS_ST/1
  Bus Selector4/4 -> Bus Creator1/4  "<Index_un8>"

== system LM_TOS_0115/adapter2/Lane_1/Subsystem1 ==
  <LANE_1_TARGETOBJECT_0_ST> : Inport
  Bus Creator1 : BusCreator  Inputs=9  OutDataTypeStr=Bus: TARGETOBJECT  NonVirtualBus=on
  Bus Selector4 : BusSelector  OutputSignals=dis2EgoLaneCenter,TTC_f,ID_un8,Index_un8,probWithinLane_arr_f_0,probWithinLane_arr_f_1,probWithinLane_arr_f_2,probWithinLane_arr_f_3,probWithinLane_arr_f_4,probCutIn_f,probCutOut_f,overlap_f,trackingTimeWithinLane_f
  Vector Concatenate : Concatenate  NumInputs=5
  TARGRTOBJECTS_ST : Outport  OutDataTypeStr=Bus: TARGETOBJECT
  wires:
  Bus Selector4/4 -> Bus Creator1/4  "<Index_un8>"
  Bus Creator1/1 -> TARGRTOBJECTS_ST/1
  Bus Selector4/3 -> Bus Creator1/3  "<ID_un8>"
  Vector Concatenate/1 -> Bus Creator1/5
  Bus Selector4/7 -> Vector Concatenate/3  "<probWithinLane_arr_f_2>"
  Bus Selector4/1 -> Bus Creator1/1  "<dis2EgoLaneCenter>"
  Bus Selector4/13 -> Bus Creator1/9  "<trackingTimeWithinLane_f>"
  Bus Selector4/6 -> Vector Concatenate/2  "<probWithinLane_arr_f_1>"
  <LANE_1_TARGETOBJECT_0_ST>/1 -> Bus Selector4/1
  Bus Selector4/5 -> Vector Concatenate/1  "<probWithinLane_arr_f_0>"
  Bus Selector4/2 -> Bus Creator1/2  "<TTC_f>"
  Bus Selector4/9 -> Vector Concatenate/5  "<probWithinLane_arr_f_4>"
  Bus Selector4/12 -> Bus Creator1/8  "<overlap_f>"
  Bus Selector4/10 -> Bus Creator1/6  "<probCutIn_f>"
  Bus Selector4/11 -> Bus Creator1/7  "<probCutOut_f>"
  Bus Selector4/8 -> Vector Concatenate/4  "<probWithinLane_arr_f_3>"

== system LM_TOS_0115/adapter2/Lane_1/Subsystem10 ==
  <LANE_1_TARGETOBJECT_0_ST> : Inport
  Bus Creator1 : BusCreator  Inputs=7  OutDataTypeStr=Bus: SEGMENT  NonVirtualBus=on
  Bus Selector4 : BusSelector  OutputSignals=coef_arr_f_0,coef_arr_f_1,coef_arr_f_2,coef_arr_f_3,dlowerLimit_f,dupperLimit_f,numOfSegment_un8,available_b,detectedByVideo_b,quality_f
  Vector Concatenate : Concatenate  NumInputs=4
  SEGMENT_ST : Outport  OutDataTypeStr=Bus: SEGMENT
  wires:
  Bus Selector4/6 -> Bus Creator1/3  "<dupperLimit_f>"
  Bus Selector4/7 -> Bus Creator1/4  "<numOfSegment_un8>"
  Bus Selector4/8 -> Bus Creator1/5  "<available_b>"
  Bus Selector4/9 -> Bus Creator1/6  "<detectedByVideo_b>"
  Bus Selector4/10 -> Bus Creator1/7  "<quality_f>"
  Bus Selector4/5 -> Bus Creator1/2  "<dlowerLimit_f>"
  Vector Concatenate/1 -> Bus Creator1/1
  Bus Selector4/4 -> Vector Concatenate/4  "<coef_arr_f_3>"
  Bus Selector4/3 -> Vector Concatenate/3  "<coef_arr_f_2>"
  Bus Selector4/1 -> Vector Concatenate/1  "<coef_arr_f_0>"
  Bus Selector4/2 -> Vector Concatenate/2  "<coef_arr_f_1>"
  <LANE_1_TARGETOBJECT_0_ST>/1 -> Bus Selector4/1
  Bus Creator1/1 -> SEGMENT_ST/1

== system LM_TOS_0115/adapter2/Lane_1/Subsystem11 ==
  <LANE_1_TARGETOBJECT_0_ST> : Inport
  Bus Creator1 : BusCreator  Inputs=7  OutDataTypeStr=Bus: SEGMENT  NonVirtualBus=on
  Bus Selector4 : BusSelector  OutputSignals=coef_arr_f_0,coef_arr_f_1,coef_arr_f_2,coef_arr_f_3,dlowerLimit_f,dupperLimit_f,numOfSegment_un8,available_b,detectedByVideo_b,quality_f
  Vector Concatenate : Concatenate  NumInputs=4
  SEGMENT_ST : Outport  OutDataTypeStr=Bus: SEGMENT
  wires:
  Bus Creator1/1 -> SEGMENT_ST/1
  <LANE_1_TARGETOBJECT_0_ST>/1 -> Bus Selector4/1
  Bus Selector4/2 -> Vector Concatenate/2  "<coef_arr_f_1>"
  Bus Selector4/1 -> Vector Concatenate/1  "<coef_arr_f_0>"
  Bus Selector4/3 -> Vector Concatenate/3  "<coef_arr_f_2>"
  Bus Selector4/4 -> Vector Concatenate/4  "<coef_arr_f_3>"
  Vector Concatenate/1 -> Bus Creator1/1
  Bus Selector4/5 -> Bus Creator1/2  "<dlowerLimit_f>"
  Bus Selector4/10 -> Bus Creator1/7  "<quality_f>"
  Bus Selector4/9 -> Bus Creator1/6  "<detectedByVideo_b>"
  Bus Selector4/8 -> Bus Creator1/5  "<available_b>"
  Bus Selector4/7 -> Bus Creator1/4  "<numOfSegment_un8>"
  Bus Selector4/6 -> Bus Creator1/3  "<dupperLimit_f>"

== system LM_TOS_0115/adapter2/Lane_1/Subsystem12 ==
  <LANE_1_TARGETOBJECT_0_ST> : Inport
  Bus Creator1 : BusCreator  Inputs=7  OutDataTypeStr=Bus: SEGMENT  NonVirtualBus=on
  Bus Selector4 : BusSelector  OutputSignals=coef_arr_f_0,coef_arr_f_1,coef_arr_f_2,coef_arr_f_3,dlowerLimit_f,dupperLimit_f,numOfSegment_un8,available_b,detectedByVideo_b,quality_f
  Vector Concatenate : Concatenate  NumInputs=4
  SEGMENT_ST : Outport  OutDataTypeStr=Bus: SEGMENT
  wires:
  Bus Selector4/6 -> Bus Creator1/3  "<dupperLimit_f>"
  Bus Selector4/7 -> Bus Creator1/4  "<numOfSegment_un8>"
  Bus Selector4/8 -> Bus Creator1/5  "<available_b>"
  Bus Selector4/9 -> Bus Creator1/6  "<detectedByVideo_b>"
  Bus Selector4/10 -> Bus Creator1/7  "<quality_f>"
  Bus Selector4/5 -> Bus Creator1/2  "<dlowerLimit_f>"
  Vector Concatenate/1 -> Bus Creator1/1
  Bus Selector4/4 -> Vector Concatenate/4  "<coef_arr_f_3>"
  Bus Selector4/3 -> Vector Concatenate/3  "<coef_arr_f_2>"
  Bus Selector4/1 -> Vector Concatenate/1  "<coef_arr_f_0>"
  Bus Selector4/2 -> Vector Concatenate/2  "<coef_arr_f_1>"
  <LANE_1_TARGETOBJECT_0_ST>/1 -> Bus Selector4/1
  Bus Creator1/1 -> SEGMENT_ST/1

== system LM_TOS_0115/adapter2/Lane_1/Subsystem13 ==
  <LANE_1_TARGETOBJECT_0_ST> : Inport
  Bus Creator1 : BusCreator  Inputs=7  OutDataTypeStr=Bus: SEGMENT  NonVirtualBus=on
  Bus Selector4 : BusSelector  OutputSignals=coef_arr_f_0,coef_arr_f_1,coef_arr_f_2,coef_arr_f_3,dlowerLimit_f,dupperLimit_f,numOfSegment_un8,available_b,detectedByVideo_b,quality_f
  Vector Concatenate : Concatenate  NumInputs=4
  SEGMENT_ST : Outport  OutDataTypeStr=Bus: SEGMENT
  wires:
  Bus Creator1/1 -> SEGMENT_ST/1
  <LANE_1_TARGETOBJECT_0_ST>/1 -> Bus Selector4/1
  Bus Selector4/2 -> Vector Concatenate/2  "<coef_arr_f_1>"
  Bus Selector4/1 -> Vector Concatenate/1  "<coef_arr_f_0>"
  Bus Selector4/3 -> Vector Concatenate/3  "<coef_arr_f_2>"
  Bus Selector4/4 -> Vector Concatenate/4  "<coef_arr_f_3>"
  Vector Concatenate/1 -> Bus Creator1/1
  Bus Selector4/5 -> Bus Creator1/2  "<dlowerLimit_f>"
  Bus Selector4/10 -> Bus Creator1/7  "<quality_f>"
  Bus Selector4/9 -> Bus Creator1/6  "<detectedByVideo_b>"
  Bus Selector4/8 -> Bus Creator1/5  "<available_b>"
  Bus Selector4/7 -> Bus Creator1/4  "<numOfSegment_un8>"
  Bus Selector4/6 -> Bus Creator1/3  "<dupperLimit_f>"

== system LM_TOS_0115/adapter2/Lane_1/Subsystem14 ==
  <LANE_1_TARGETOBJECT_0_ST> : Inport
  Bus Creator1 : BusCreator  Inputs=7  OutDataTypeStr=Bus: SEGMENT  NonVirtualBus=on
  Bus Selector4 : BusSelector  OutputSignals=coef_arr_f_0,coef_arr_f_1,coef_arr_f_2,coef_arr_f_3,dlowerLimit_f,dupperLimit_f,numOfSegment_un8,available_b,detectedByVideo_b,quality_f
  Vector Concatenate : Concatenate  NumInputs=4
  SEGMENT_ST : Outport  OutDataTypeStr=Bus: SEGMENT
  wires:
  Bus Selector4/6 -> Bus Creator1/3  "<dupperLimit_f>"
  Bus Selector4/7 -> Bus Creator1/4  "<numOfSegment_un8>"
  Bus Selector4/8 -> Bus Creator1/5  "<available_b>"
  Bus Selector4/9 -> Bus Creator1/6  "<detectedByVideo_b>"
  Bus Selector4/10 -> Bus Creator1/7  "<quality_f>"
  Bus Selector4/5 -> Bus Creator1/2  "<dlowerLimit_f>"
  Vector Concatenate/1 -> Bus Creator1/1
  Bus Selector4/4 -> Vector Concatenate/4  "<coef_arr_f_3>"
  Bus Selector4/3 -> Vector Concatenate/3  "<coef_arr_f_2>"
  Bus Selector4/1 -> Vector Concatenate/1  "<coef_arr_f_0>"
  Bus Selector4/2 -> Vector Concatenate/2  "<coef_arr_f_1>"
  <LANE_1_TARGETOBJECT_0_ST>/1 -> Bus Selector4/1
  Bus Creator1/1 -> SEGMENT_ST/1

== system LM_TOS_0115/adapter2/Lane_1/Subsystem15 ==
  <LANE_1_TARGETOBJECT_0_ST> : Inport
  Bus Creator1 : BusCreator  Inputs=7  OutDataTypeStr=Bus: SEGMENT  NonVirtualBus=on
  Bus Selector4 : BusSelector  OutputSignals=coef_arr_f_0,coef_arr_f_1,coef_arr_f_2,coef_arr_f_3,dlowerLimit_f,dupperLimit_f,numOfSegment_un8,available_b,detectedByVideo_b,quality_f
  Vector Concatenate : Concatenate  NumInputs=4
  SEGMENT_ST : Outport  OutDataTypeStr=Bus: SEGMENT
  wires:
  Bus Creator1/1 -> SEGMENT_ST/1
  <LANE_1_TARGETOBJECT_0_ST>/1 -> Bus Selector4/1
  Bus Selector4/2 -> Vector Concatenate/2  "<coef_arr_f_1>"
  Bus Selector4/1 -> Vector Concatenate/1  "<coef_arr_f_0>"
  Bus Selector4/3 -> Vector Concatenate/3  "<coef_arr_f_2>"
  Bus Selector4/4 -> Vector Concatenate/4  "<coef_arr_f_3>"
  Vector Concatenate/1 -> Bus Creator1/1
  Bus Selector4/5 -> Bus Creator1/2  "<dlowerLimit_f>"
  Bus Selector4/10 -> Bus Creator1/7  "<quality_f>"
  Bus Selector4/9 -> Bus Creator1/6  "<detectedByVideo_b>"
  Bus Selector4/8 -> Bus Creator1/5  "<available_b>"
  Bus Selector4/7 -> Bus Creator1/4  "<numOfSegment_un8>"
  Bus Selector4/6 -> Bus Creator1/3  "<dupperLimit_f>"

== system LM_TOS_0115/adapter2/Lane_1/Subsystem2 ==
  <LANE_1_TARGETOBJECT_0_ST> : Inport
  Bus Creator1 : BusCreator  Inputs=9  OutDataTypeStr=Bus: TARGETOBJECT  NonVirtualBus=on
  Bus Selector4 : BusSelector  OutputSignals=dis2EgoLaneCenter,TTC_f,ID_un8,Index_un8,probWithinLane_arr_f_0,probWithinLane_arr_f_1,probWithinLane_arr_f_2,probWithinLane_arr_f_3,probWithinLane_arr_f_4,probCutIn_f,probCutOut_f,overlap_f,trackingTimeWithinLane_f
  Vector Concatenate : Concatenate  NumInputs=5
  TARGRTOBJECTS_ST : Outport  OutDataTypeStr=Bus: TARGETOBJECT
  wires:
  Bus Selector4/8 -> Vector Concatenate/4  "<probWithinLane_arr_f_3>"
  Bus Selector4/11 -> Bus Creator1/7  "<probCutOut_f>"
  Bus Selector4/10 -> Bus Creator1/6  "<probCutIn_f>"
  Bus Selector4/12 -> Bus Creator1/8  "<overlap_f>"
  Bus Selector4/9 -> Vector Concatenate/5  "<probWithinLane_arr_f_4>"
  Bus Selector4/2 -> Bus Creator1/2  "<TTC_f>"
  Bus Selector4/5 -> Vector Concatenate/1  "<probWithinLane_arr_f_0>"
  <LANE_1_TARGETOBJECT_0_ST>/1 -> Bus Selector4/1
  Bus Selector4/6 -> Vector Concatenate/2  "<probWithinLane_arr_f_1>"
  Bus Selector4/13 -> Bus Creator1/9  "<trackingTimeWithinLane_f>"
  Bus Selector4/1 -> Bus Creator1/1  "<dis2EgoLaneCenter>"
  Bus Selector4/7 -> Vector Concatenate/3  "<probWithinLane_arr_f_2>"
  Vector Concatenate/1 -> Bus Creator1/5
  Bus Selector4/3 -> Bus Creator1/3  "<ID_un8>"
  Bus Creator1/1 -> TARGRTOBJECTS_ST/1
  Bus Selector4/4 -> Bus Creator1/4  "<Index_un8>"

== system LM_TOS_0115/adapter2/Lane_1/Subsystem3 ==
  <LANE_1_TARGETOBJECT_0_ST> : Inport
  Bus Creator1 : BusCreator  Inputs=9  OutDataTypeStr=Bus: TARGETOBJECT  NonVirtualBus=on
  Bus Selector4 : BusSelector  OutputSignals=dis2EgoLaneCenter,TTC_f,ID_un8,Index_un8,probWithinLane_arr_f_0,probWithinLane_arr_f_1,probWithinLane_arr_f_2,probWithinLane_arr_f_3,probWithinLane_arr_f_4,probCutIn_f,probCutOut_f,overlap_f,trackingTimeWithinLane_f
  Vector Concatenate : Concatenate  NumInputs=5
  TARGRTOBJECTS_ST : Outport  OutDataTypeStr=Bus: TARGETOBJECT
  wires:
  Bus Selector4/4 -> Bus Creator1/4  "<Index_un8>"
  Bus Creator1/1 -> TARGRTOBJECTS_ST/1
  Bus Selector4/3 -> Bus Creator1/3  "<ID_un8>"
  Vector Concatenate/1 -> Bus Creator1/5
  Bus Selector4/7 -> Vector Concatenate/3  "<probWithinLane_arr_f_2>"
  Bus Selector4/1 -> Bus Creator1/1  "<dis2EgoLaneCenter>"
  Bus Selector4/13 -> Bus Creator1/9  "<trackingTimeWithinLane_f>"
  Bus Selector4/6 -> Vector Concatenate/2  "<probWithinLane_arr_f_1>"
  <LANE_1_TARGETOBJECT_0_ST>/1 -> Bus Selector4/1
  Bus Selector4/5 -> Vector Concatenate/1  "<probWithinLane_arr_f_0>"
  Bus Selector4/2 -> Bus Creator1/2  "<TTC_f>"
  Bus Selector4/9 -> Vector Concatenate/5  "<probWithinLane_arr_f_4>"
  Bus Selector4/12 -> Bus Creator1/8  "<overlap_f>"
  Bus Selector4/10 -> Bus Creator1/6  "<probCutIn_f>"
  Bus Selector4/11 -> Bus Creator1/7  "<probCutOut_f>"
  Bus Selector4/8 -> Vector Concatenate/4  "<probWithinLane_arr_f_3>"

== system LM_TOS_0115/adapter2/Lane_1/Subsystem4 ==
  <LANE_1_TARGETOBJECT_0_ST> : Inport
  Bus Creator1 : BusCreator  Inputs=9  OutDataTypeStr=Bus: TARGETOBJECT  NonVirtualBus=on
  Bus Selector4 : BusSelector  OutputSignals=dis2EgoLaneCenter,TTC_f,ID_un8,Index_un8,probWithinLane_arr_f_0,probWithinLane_arr_f_1,probWithinLane_arr_f_2,probWithinLane_arr_f_3,probWithinLane_arr_f_4,probCutIn_f,probCutOut_f,overlap_f,trackingTimeWithinLane_f
  Vector Concatenate : Concatenate  NumInputs=5
  TARGRTOBJECTS_ST : Outport  OutDataTypeStr=Bus: TARGETOBJECT
  wires:
  Bus Selector4/8 -> Vector Concatenate/4  "<probWithinLane_arr_f_3>"
  Bus Selector4/11 -> Bus Creator1/7  "<probCutOut_f>"
  Bus Selector4/10 -> Bus Creator1/6  "<probCutIn_f>"
  Bus Selector4/12 -> Bus Creator1/8  "<overlap_f>"
  Bus Selector4/9 -> Vector Concatenate/5  "<probWithinLane_arr_f_4>"
  Bus Selector4/2 -> Bus Creator1/2  "<TTC_f>"
  Bus Selector4/5 -> Vector Concatenate/1  "<probWithinLane_arr_f_0>"
  <LANE_1_TARGETOBJECT_0_ST>/1 -> Bus Selector4/1
  Bus Selector4/6 -> Vector Concatenate/2  "<probWithinLane_arr_f_1>"
  Bus Selector4/13 -> Bus Creator1/9  "<trackingTimeWithinLane_f>"
  Bus Selector4/1 -> Bus Creator1/1  "<dis2EgoLaneCenter>"
  Bus Selector4/7 -> Vector Concatenate/3  "<probWithinLane_arr_f_2>"
  Vector Concatenate/1 -> Bus Creator1/5
  Bus Selector4/3 -> Bus Creator1/3  "<ID_un8>"
  Bus Creator1/1 -> TARGRTOBJECTS_ST/1
  Bus Selector4/4 -> Bus Creator1/4  "<Index_un8>"

== system LM_TOS_0115/adapter2/Lane_1/Subsystem5 ==
  <LANE_1_TARGETOBJECT_0_ST> : Inport
  Bus Creator1 : BusCreator  Inputs=9  OutDataTypeStr=Bus: TARGETOBJECT  NonVirtualBus=on
  Bus Selector4 : BusSelector  OutputSignals=dis2EgoLaneCenter,TTC_f,ID_un8,Index_un8,probWithinLane_arr_f_0,probWithinLane_arr_f_1,probWithinLane_arr_f_2,probWithinLane_arr_f_3,probWithinLane_arr_f_4,probCutIn_f,probCutOut_f,overlap_f,trackingTimeWithinLane_f
  Vector Concatenate : Concatenate  NumInputs=5
  TARGRTOBJECTS_ST : Outport  OutDataTypeStr=Bus: TARGETOBJECT
  wires:
  Bus Selector4/4 -> Bus Creator1/4  "<Index_un8>"
  Bus Creator1/1 -> TARGRTOBJECTS_ST/1
  Bus Selector4/3 -> Bus Creator1/3  "<ID_un8>"
  Vector Concatenate/1 -> Bus Creator1/5
  Bus Selector4/7 -> Vector Concatenate/3  "<probWithinLane_arr_f_2>"
  Bus Selector4/1 -> Bus Creator1/1  "<dis2EgoLaneCenter>"
  Bus Selector4/13 -> Bus Creator1/9  "<trackingTimeWithinLane_f>"
  Bus Selector4/6 -> Vector Concatenate/2  "<probWithinLane_arr_f_1>"
  <LANE_1_TARGETOBJECT_0_ST>/1 -> Bus Selector4/1
  Bus Selector4/5 -> Vector Concatenate/1  "<probWithinLane_arr_f_0>"
  Bus Selector4/2 -> Bus Creator1/2  "<TTC_f>"
  Bus Selector4/9 -> Vector Concatenate/5  "<probWithinLane_arr_f_4>"
  Bus Selector4/12 -> Bus Creator1/8  "<overlap_f>"
  Bus Selector4/10 -> Bus Creator1/6  "<probCutIn_f>"
  Bus Selector4/11 -> Bus Creator1/7  "<probCutOut_f>"
  Bus Selector4/8 -> Vector Concatenate/4  "<probWithinLane_arr_f_3>"

== system LM_TOS_0115/adapter2/Lane_1/Subsystem6 ==
  <LANE_1_TARGETOBJECT_0_ST> : Inport
  Bus Creator1 : BusCreator  Inputs=9  OutDataTypeStr=Bus: TARGETOBJECT  NonVirtualBus=on
  Bus Selector4 : BusSelector  OutputSignals=dis2EgoLaneCenter,TTC_f,ID_un8,Index_un8,probWithinLane_arr_f_0,probWithinLane_arr_f_1,probWithinLane_arr_f_2,probWithinLane_arr_f_3,probWithinLane_arr_f_4,probCutIn_f,probCutOut_f,overlap_f,trackingTimeWithinLane_f
  Vector Concatenate : Concatenate  NumInputs=5
  TARGRTOBJECTS_ST : Outport  OutDataTypeStr=Bus: TARGETOBJECT
  wires:
  Bus Selector4/8 -> Vector Concatenate/4  "<probWithinLane_arr_f_3>"
  Bus Selector4/11 -> Bus Creator1/7  "<probCutOut_f>"
  Bus Selector4/10 -> Bus Creator1/6  "<probCutIn_f>"
  Bus Selector4/12 -> Bus Creator1/8  "<overlap_f>"
  Bus Selector4/9 -> Vector Concatenate/5  "<probWithinLane_arr_f_4>"
  Bus Selector4/2 -> Bus Creator1/2  "<TTC_f>"
  Bus Selector4/5 -> Vector Concatenate/1  "<probWithinLane_arr_f_0>"
  <LANE_1_TARGETOBJECT_0_ST>/1 -> Bus Selector4/1
  Bus Selector4/6 -> Vector Concatenate/2  "<probWithinLane_arr_f_1>"
  Bus Selector4/13 -> Bus Creator1/9  "<trackingTimeWithinLane_f>"
  Bus Selector4/1 -> Bus Creator1/1  "<dis2EgoLaneCenter>"
  Bus Selector4/7 -> Vector Concatenate/3  "<probWithinLane_arr_f_2>"
  Vector Concatenate/1 -> Bus Creator1/5
  Bus Selector4/3 -> Bus Creator1/3  "<ID_un8>"
  Bus Creator1/1 -> TARGRTOBJECTS_ST/1
  Bus Selector4/4 -> Bus Creator1/4  "<Index_un8>"

== system LM_TOS_0115/adapter2/Lane_1/Subsystem7 ==
  <LANE_1_TARGETOBJECT_0_ST> : Inport
  Bus Creator1 : BusCreator  Inputs=9  OutDataTypeStr=Bus: TARGETOBJECT  NonVirtualBus=on
  Bus Selector4 : BusSelector  OutputSignals=dis2EgoLaneCenter,TTC_f,ID_un8,Index_un8,probWithinLane_arr_f_0,probWithinLane_arr_f_1,probWithinLane_arr_f_2,probWithinLane_arr_f_3,probWithinLane_arr_f_4,probCutIn_f,probCutOut_f,overlap_f,trackingTimeWithinLane_f
  Vector Concatenate : Concatenate  NumInputs=5
  TARGRTOBJECTS_ST : Outport  OutDataTypeStr=Bus: TARGETOBJECT
  wires:
  Bus Selector4/4 -> Bus Creator1/4  "<Index_un8>"
  Bus Creator1/1 -> TARGRTOBJECTS_ST/1
  Bus Selector4/3 -> Bus Creator1/3  "<ID_un8>"
  Vector Concatenate/1 -> Bus Creator1/5
  Bus Selector4/7 -> Vector Concatenate/3  "<probWithinLane_arr_f_2>"
  Bus Selector4/1 -> Bus Creator1/1  "<dis2EgoLaneCenter>"
  Bus Selector4/13 -> Bus Creator1/9  "<trackingTimeWithinLane_f>"
  Bus Selector4/6 -> Vector Concatenate/2  "<probWithinLane_arr_f_1>"
  <LANE_1_TARGETOBJECT_0_ST>/1 -> Bus Selector4/1
  Bus Selector4/5 -> Vector Concatenate/1  "<probWithinLane_arr_f_0>"
  Bus Selector4/2 -> Bus Creator1/2  "<TTC_f>"
  Bus Selector4/9 -> Vector Concatenate/5  "<probWithinLane_arr_f_4>"
  Bus Selector4/12 -> Bus Creator1/8  "<overlap_f>"
  Bus Selector4/10 -> Bus Creator1/6  "<probCutIn_f>"
  Bus Selector4/11 -> Bus Creator1/7  "<probCutOut_f>"
  Bus Selector4/8 -> Vector Concatenate/4  "<probWithinLane_arr_f_3>"
